simulink model "SetResetOut_tmp"  (Simulink 8.3)
settings: Solver=FixedStepDiscrete  StartTime=0.0  StopTime=10000.0  RelTol=1e-3
settings Model: Creator=scaife  LastModifiedBy=bourbouh  CovSFcnEnable=on  ExtModeAutoUpdateStatusClock=off
settings DataIOCC: SignalLoggingName=sigsOut
settings DebuggingCC: SaveWithParameterizedLinksMsg=none  SignalResolutionControl=TryResolveAllWithWarning  SolverPrmCheckMsg=none  MultiTaskDSMMsg=warning  MultiTaskCondExecSysMsg=none  FrameProcessingCompatibilityMsg=error  StateNameClashWarn=none  StrictBusMsg=None
settings HardwareCC: TargetUnknown=on
settings SFSimCC: SimParseCustomCode=off
settings GRTTargetCC: GeneratePreprocessorConditionals=Use local settings

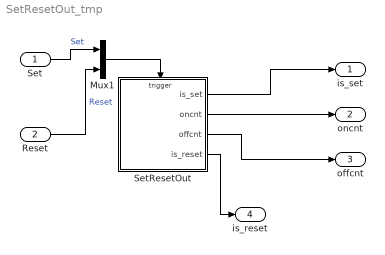
== system SetResetOut_tmp ==
  Set : Inport
  Reset : Inport  Port=2
  Mux1 : Mux  Inputs=2
  SetResetOut : Stateflow chart  TreatAsAtomicUnit=on
      settings: PermitHierarchicalResolution=ParametersOnly
  is_set : Outport
  oncnt : Outport  Port=2
  offcnt : Outport  Port=3
  is_reset : Outport  Port=4
  wires:
  Mux1/1 -> SetResetOut/Trigger
  Set/1 -> Mux1/1  "Set"
  Reset/1 -> Mux1/2  "Reset"
  SetResetOut/4(is_reset) -> is_reset/1
  SetResetOut/3(offcnt) -> offcnt/1
  SetResetOut/2(oncnt) -> oncnt/1
  SetResetOut/1(is_set) -> is_set/1

== stateflow chart SetResetOut ==
  state On/
    en: is_set=1; oncnt++;
    du: oncnt++;
    ex: is_reset=1;
  state Off/
    en: is_set=2; offcnt++;
    du: offcnt++;
    ex: is_reset=2;
  (default) -> Off
  Off -> On : Set
  On -> Off : Reset
  data: is_set output int32; oncnt output int32; offcnt output int32; is_reset output int32
  events: Set input EITHER_EDGE_EVENT; Reset input EITHER_EDGE_EVENT
